simulink model "Open_System"  (R2021b)
settings: Solver=VariableStepAuto  StartTime=0.0  StopTime=10.0  RelTol=1e-3
settings Model: Creator=yyfyyf  LastModifiedBy=yyfyyf

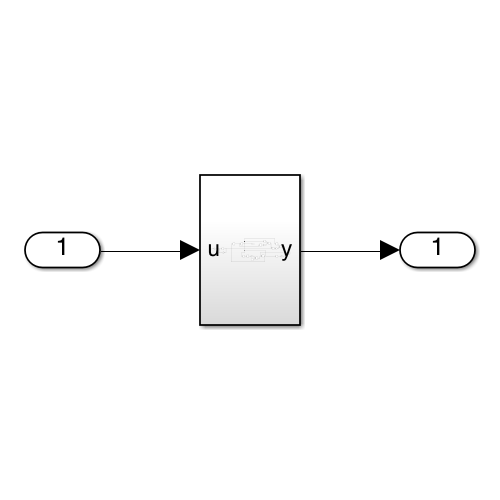
[thumbnail: Simulink's stored preview of the top-level diagram]
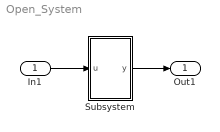
== system Open_System ==
  In1 : Inport
  Subsystem : Subsystem
  Out1 : Outport
  wires:
  Subsystem/1(y) -> Out1/1
  In1/1 -> Subsystem/1(u)

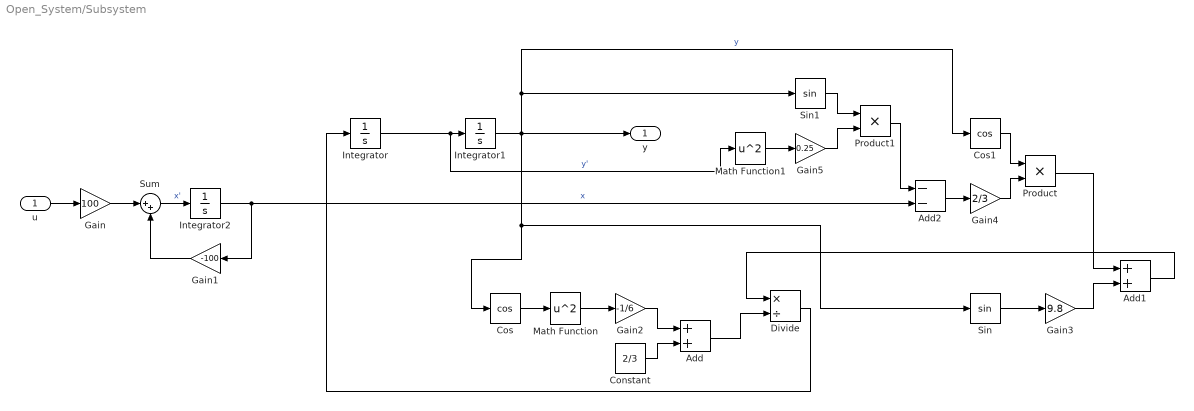
== system Open_System/Subsystem ==
  u : Inport
  Add : Sum
  Add1 : Sum
  Add2 : Sum  Inputs=--
  Constant : Constant  Value=2/3
  Cos : Trigonometry  Operator=cos
  Cos1 : Trigonometry  Operator=cos
  Divide : Product  Inputs=*/
  Gain : Gain  Gain=100
  Gain1 : Gain  Gain=-100
  Gain2 : Gain  Gain=-1/6
  Gain3 : Gain  Gain=9.8
  Gain4 : Gain  Gain=2/3
  Gain5 : Gain  Gain=0.25
  Integrator : Integrator
  Integrator1 : Integrator  InitialCondition=0.1
  Integrator2 : Integrator
  Math Function : Math  Operator=square  SaturateOnIntegerOverflow=on
  Math Function1 : Math  Operator=square  SaturateOnIntegerOverflow=on
  Product : Product
  Product1 : Product
  Sin : Trigonometry
  Sin1 : Trigonometry
  Sum : Sum  Inputs=|++
  y : Outport
  wires:
  Cos/1 -> Math Function/1
  Integrator1/1 -> Cos1/1, Sin1/1, y/1, Cos/1, Sin/1  "y"
  Constant/1 -> Add/2
  Add2/1 -> Gain4/1
  u/1 -> Gain/1
  Sum/1 -> Integrator2/1  "x'"
  Math Function1/1 -> Gain5/1
  Sin1/1 -> Product1/1
  Gain1/1 -> Sum/2
  Sin/1 -> Gain3/1
  Gain5/1 -> Product1/2
  Product1/1 -> Add2/1
  Product/1 -> Add1/1
  Add/1 -> Divide/2
  Add1/1 -> Divide/1
  Integrator/1 -> Math Function1/1, Integrator1/1  "y'"
  Gain/1 -> Sum/1
  Gain2/1 -> Add/1
  Divide/1 -> Integrator/1
  Integrator2/1 -> Gain1/1, Add2/2  "x"
  Cos1/1 -> Product/1
  Gain4/1 -> Product/2
  Math Function/1 -> Gain2/1
  Gain3/1 -> Add1/2
